simulink model "said2"  (R2018a)
settings: Solver=ode45  StartTime=0.0  StopTime=100  RelTol=1e-3  EnableMultiTasking=on
settings Model: Creator=SAITFASKA  LastModifiedBy=admin
settings DataIOCC: LimitDataPoints=on  SaveFormat=Array
settings OptimizationCC: LifeSpan=inf
settings DebuggingCC: UnderspecifiedInitializationDetection=Classic  MergeDetectMultiDrivingBlocksExec=none  SolverPrmCheckMsg=warning  StateNameClashWarn=warning  SFUnexpectedBacktrackingDiag=warning  SFNoUnconditionalDefaultTransitionDiag=warning  SFExecutionAtInitializationDiag=none
settings HardwareCC: ProdBitPerPointer=32  ProdBitPerSizeT=32  ProdBitPerPtrDiffT=32  ProdLargestAtomicFloat=None  ProdIntDivRoundTo=Undefined  ProdEndianess=Unspecified  ProdWordSize=32  ProdHWDeviceType=32-bit Generic
settings ModelReferenceCC: PropagateSignalLabelsOutOfModel=off
settings CodeAppCC: StateflowObjectComments=on
settings GRTTargetCC: TargetLangStandard=C89/C90 (ANSI)  GeneratePreprocessorConditionals=Disable all
settings ConfigComp: CovMetricSettings=dw  CovHtmlReporting=on  CovSaveCumulativeToWorkspaceVar=on  CovSaveSingleToWorkspaceVar=on  CovExternalEMLEnable=off

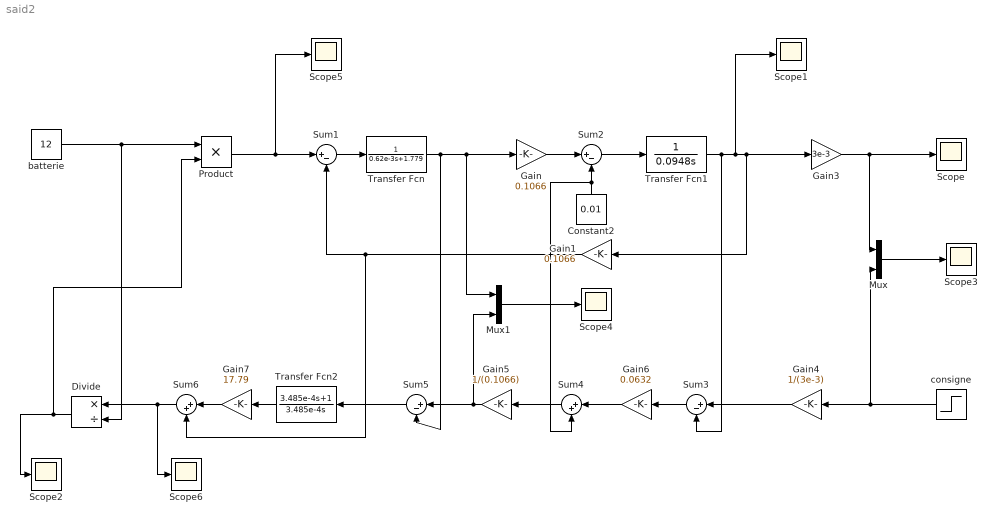
== system said2 ==
  Constant2 : Constant  Value=0.01
  Divide : Product  Inputs=*/
  Gain : Gain  Gain=0.1066
  Gain1 : Gain  Gain=0.1066
  Gain3 : Gain  Gain=3e-3
  Gain4 : Gain  Gain=1/(3e-3)
  Gain5 : Gain  Gain=1/(0.1066)
  Gain6 : Gain  Gain=0.0632
  Gain7 : Gain  Gain=17.79
  Mux : Mux  Inputs=2
  Mux1 : Mux  Inputs=2
  Product : Product
  Scope{,1..6} (7 alike) : Scope
  Sum{1..3,5} (4 alike) : Sum  Inputs=|+-
  Sum4 : Sum  Inputs=|++
  Sum6 : Sum  Inputs=|++
  Transfer Fcn : TransferFcn  Denominator="[0.62e-3  1.779]"
  Transfer Fcn1 : TransferFcn  Denominator=[ 0.0948 0]
  Transfer Fcn2 : TransferFcn  Numerator=[3.485e-4 1]  Denominator=[3.485e-4 0]
  batterie : Constant  Value=12
  consigne : Step  Time=0  After=1.3  SampleTime=0
  wires:
  Product/1 -> Scope5/1, Sum1/1
  Gain/1 -> Sum2/1
  consigne/1 -> Mux/2, Gain4/1
  Gain4/1 -> Sum3/1
  Sum3/1 -> Gain6/1
  Mux/1 -> Scope3/1
  Sum2/1 -> Transfer Fcn1/1
  Gain6/1 -> Sum4/1
  Sum4/1 -> Gain5/1
  Gain5/1 -> Sum5/1, Mux1/2
  Sum5/1 -> Transfer Fcn2/1
  Transfer Fcn2/1 -> Gain7/1
  Mux1/1 -> Scope4/1
  Gain7/1 -> Sum6/1
  Divide/1 -> Scope2/1, Product/2
  Sum1/1 -> Transfer Fcn/1
  Sum6/1 -> Divide/1, Scope6/1
  Gain1/1 -> Sum6/2, Sum1/2
  Transfer Fcn1/1 -> Sum3/2, Scope1/1, Gain3/1, Gain1/1
  Gain3/1 -> Mux/1, Scope/1
  Constant2/1 -> Sum4/2, Sum2/2
  Transfer Fcn/1 -> Sum5/2, Mux1/1, Gain/1
  batterie/1 -> Divide/2, Product/1
